simulink library "purePursuitWithWarpingCtrl_cl"  (R2018a)
settings: Solver=VariableStepAuto  StartTime=0.0  StopTime=10.0  RelTol=1e-3
values from neighbouring files (symbols this model uses):
  numberOfLaps_none = 5    [purePursuitWithWarpingCtrl_cl_init.m]
libraries: simulink x1, headingSetpointwithWarpingCalculation_cl x1, lapCounter_ul x1, runningAverage_cl x1
settings Model: Creator=mcobb  LastModifiedBy=mcobb

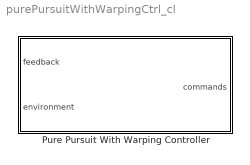
== system purePursuitWithWarpingCtrl_cl ==
  Pure Pursuit With Warping Controller : Subsystem  VariantControl=VSS_PUREPURSUITWITHWARPING_CTRL

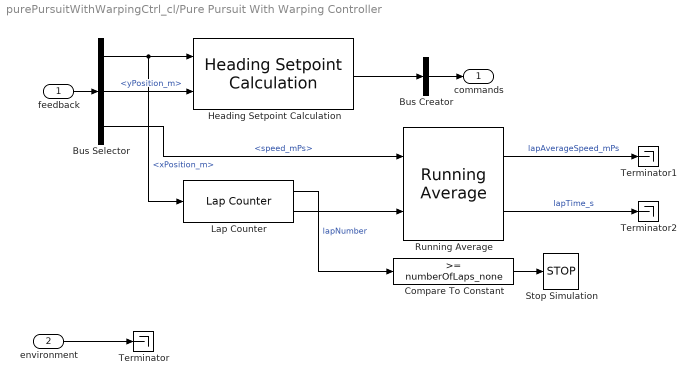
== system purePursuitWithWarpingCtrl_cl/Pure Pursuit With Warping Controller ==
  feedback : Inport
  environment : Inport  Port=2
  Bus Creator : BusCreator  Inputs=1
  Bus Selector : BusSelector  OutputSignals=xPosition_m,yPosition_m,speed_mPs
  Compare To Constant : simulink/Logic and Bit Operations/Compare To Constant  relop=>=  const=numberOfLaps_none  OutDataTypeStr=boolean
  Heading Setpoint Calculation : headingSetpointwithWarpingCalculation_cl/Heading Setpoint Calculation
  Lap Counter : lapCounter_ul/Lap Counter
  Running Average : runningAverage_cl/Running Average
  Stop Simulation : Stop
  Terminator : Terminator
  Terminator1 : Terminator
  Terminator2 : Terminator
  commands : Outport
  wires:
  feedback/1 -> Bus Selector/1
  Bus Selector/1 -> Lap Counter/1, Heading Setpoint Calculation/1  "<xPosition_m>"
  Bus Selector/2 -> Heading Setpoint Calculation/2  "<yPosition_m>"
  environment/1 -> Terminator/1
  Heading Setpoint Calculation/1 -> Bus Creator/1
  Bus Creator/1 -> commands/1
  Lap Counter/1 -> Compare To Constant/1  "lapNumber"
  Compare To Constant/1 -> Stop Simulation/1
  Bus Selector/3 -> Running Average/1  "<speed_mPs>"
  Running Average/1 -> Terminator1/1  "lapAverageSpeed_mPs"
  Lap Counter/2 -> Running Average/2
  Running Average/2 -> Terminator2/1  "lapTime_s"
